simulink model "power_transfo3ph"  (Simulink 6.0)
settings: Solver=ode15s  SolverMode=SingleTasking  StartTime=0.0  StopTime=0.5  RelTol=1e-3  AbsTol=1e-2
libraries: powerlib x16, powerlib_extras x1
settings Model: Creator=patrice  LastModifiedBy=batserve  ExtModeTrigMode=oneshot  ExtModeArmWhenConnect=off  ExtModeAutoUpdateStatusClock=off
settings DataIOCC: LimitDataPoints=off  SignalLoggingName=sigsOut
settings OptimizationCC: BooleanDataType=off
settings DebuggingCC: SolverPrmCheckMsg=none  IntegerOverflowMsg=none
settings HardwareCC: TargetUnknown=on
settings RTWCC: TemplateMakefile=grt_unix.tmf

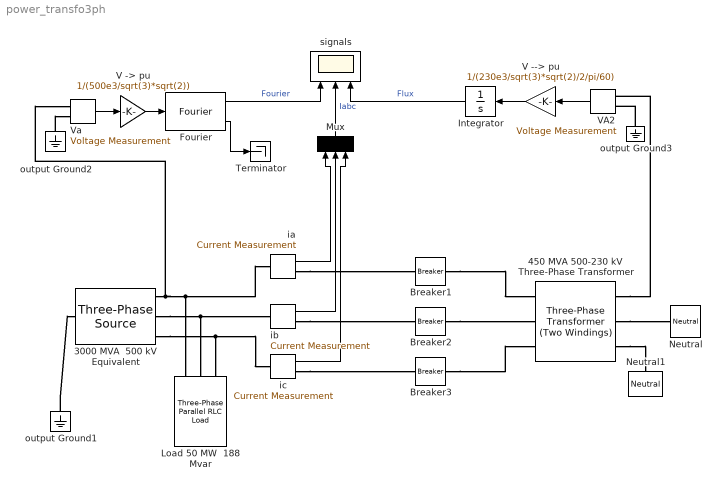
== system power_transfo3ph ==
  3000 MVA  500 kV Equivalent : powerlib/Electrical Sources/Three-Phase Source  Voltage=500e3  PhaseAngle=0  Frequency=60  InternalConnection=Yn  SpecifyImpedance=off  Resistance=5.55  Inductance=0.221  ShortCircuitLevel=100e6  BaseVoltage=25e3  XRratio=7
  450 MVA 500-230 kV Three-Phase Transformer : powerlib/Elements/Three-Phase Transformer (Two Windings)  NominalPower=[ 450e6 60 ]  Winding1Connection=Yg  Winding1=[ 500e3 0.002 0.08 ]  Winding2Connection=Yg  Winding2=[ 230e3 0.002 0.08]  SetSaturation=on  Rm=500  Lm=500  Saturation="[0 0; 0.0 1.2; 1.0  1.52]"  Hysteresis=off  DataFile='hysteresis'  SetInitialFlux=on  InitialFluxes="[0.8  -0.4  0.4]"  Measurements=None  TransfoNumber=0
  Breaker1 : powerlib/Elements/Breaker  BreakerResistance=1e-2  InitialState=0  SnubberResistance=100e6  SnubberCapacitance=inf  SwitchingTimes=.05  External=off  Measurements=None
      settings: AttributesFormatString=\n
  Breaker2 : powerlib/Elements/Breaker  BreakerResistance=1e-2  InitialState=0  SnubberResistance=100e6  SnubberCapacitance=inf  SwitchingTimes=.05  External=off  Measurements=None
      settings: AttributesFormatString=\n
  Breaker3 : powerlib/Elements/Breaker  BreakerResistance=1e-2  InitialState=0  SnubberResistance=100e6  SnubberCapacitance=inf  SwitchingTimes=.05  External=off  Measurements=None
      settings: AttributesFormatString=\n
  Fourier : powerlib_extras/Measurements/Fourier  f1=60  n=4
  Integrator : Integrator  Orientation=left  InitialCondition=0.8
  Load 50 MW  188 Mvar : powerlib/Elements/Three-Phase Parallel RLC Load  Orientation=down  PhysicalDomain=powersysdomain  SubClassName=unknown  LeftPortType=p1  RightPortType=p1  LConnTagsString=A|B|C  Configuration=Y (grounded)  NominalVoltage=500e3  NominalFrequency=60  ActivePower=50e6  InductivePower=0  CapacitivePower=188e6  Measurements=None
  Mux : Mux  Orientation=up  Inputs=3
  Neutral : powerlib/Elements/Neutral  PhysicalDomain=powersysdomain  SubClassName=unknown  LeftPortType=p1  RightPortType=p1  LConnTagsString=a  NodeNumber=991
  Neutral1 : powerlib/Elements/Neutral  Orientation=down  PhysicalDomain=powersysdomain  SubClassName=unknown  LeftPortType=p1  RightPortType=p1  LConnTagsString=a  NodeNumber=992
  Terminator : Terminator
  V --> pu : Gain  Orientation=left  Gain=1/(230e3/sqrt(3)*sqrt(2)/2/pi/60)  SaturateOnIntegerOverflow=on
  "V -> pu" : Gain  Gain=1/(500e3/sqrt(3)*sqrt(2))  SaturateOnIntegerOverflow=on
  VA2 : powerlib/Measurements/Voltage Measurement  Tag=PoWeRsYsTeMmEaSuReMeNt  Orientation=left  PhasorSimulation=off  OutputType=Magnitude  PSBequivalent=0
  Va : powerlib/Measurements/Voltage Measurement  Tag=PoWeRsYsTeMmEaSuReMeNt  PhasorSimulation=off  OutputType=Magnitude  PSBequivalent=0
  ia : powerlib/Measurements/Current Measurement  Tag=PoWeRsYsTeMmEaSuReMeNt  PhasorSimulation=off  OutputType=Magnitude  PSBequivalent=0
  ib : powerlib/Measurements/Current Measurement  Tag=PoWeRsYsTeMmEaSuReMeNt  PhasorSimulation=off  OutputType=Magnitude  PSBequivalent=0
  ic : powerlib/Measurements/Current Measurement  Tag=PoWeRsYsTeMmEaSuReMeNt  PhasorSimulation=off  OutputType=Magnitude  PSBequivalent=0
  output Ground1 : powerlib/Elements/Ground  Orientation=down  PhysicalDomain=powersysdomain  SubClassName=unknown  LeftPortType=p1  RightPortType=p1  LConnTagsString=a
  output Ground2 : powerlib/Elements/Ground  Orientation=down  PhysicalDomain=powersysdomain  SubClassName=unknown  LeftPortType=p1  RightPortType=p1  LConnTagsString=a
  output Ground3 : powerlib/Elements/Ground  Orientation=down  PhysicalDomain=powersysdomain  SubClassName=unknown  LeftPortType=p1  RightPortType=p1  LConnTagsString=a
  signals : Scope  NumInputPorts=3
      settings: Orientation=up  TimeRange=0.2  YMin=-2000~-5~-5  YMax=3000~5~5  DataFormat=Structure
  wires:
  Fourier/2 -> Terminator/1
  "V -> pu"/1 -> Fourier/1
  Fourier/1 -> signals/1  "Fourier"
  Mux/1 -> signals/2  "Iabc"
  V --> pu/1 -> Integrator/1
  Integrator/1 -> signals/3  "Flux"
  ia/1 -> Mux/1
  ib/1 -> Mux/2
  ic/1 -> Mux/3
  Va/1 -> "V -> pu"/1
  VA2/1 -> V --> pu/1
  connections:
  output Ground1/LConn1 -- 3000 MVA  500 kV Equivalent/LConn1
  3000 MVA  500 kV Equivalent/RConn3 -- Load 50 MW  188 Mvar/LConn3 -- ic/LConn1
  3000 MVA  500 kV Equivalent/RConn2 -- Load 50 MW  188 Mvar/LConn2 -- ib/LConn1
  Breaker3/RConn1 -- 450 MVA 500-230 kV Three-Phase Transformer/LConn3
  450 MVA 500-230 kV Three-Phase Transformer/RConn2 -- Neutral/LConn1
  450 MVA 500-230 kV Three-Phase Transformer/RConn3 -- Neutral1/LConn1
  ia/RConn1 -- Breaker1/LConn1
  Breaker1/RConn1 -- 450 MVA 500-230 kV Three-Phase Transformer/LConn1
  Breaker2/RConn1 -- 450 MVA 500-230 kV Three-Phase Transformer/LConn2
  ib/RConn1 -- Breaker2/LConn1
  ic/RConn1 -- Breaker3/LConn1
  output Ground2/LConn1 -- Va/LConn2
  450 MVA 500-230 kV Three-Phase Transformer/RConn1 -- VA2/LConn1
  output Ground3/LConn1 -- VA2/LConn2
  3000 MVA  500 kV Equivalent/RConn1 -- Va/LConn1 -- Load 50 MW  188 Mvar/LConn1 -- ia/LConn1
